simulink model "model"  (R2023a)
settings: Solver=VariableStepAuto  StartTime=0.0  StopTime=0.25  RelTol=1e-3
values from neighbouring files (symbols this model uses):
  Bm = 10^(-5)    (= 1e-05)    [parameter.m]
  g = 9.81    [parameter.m]
  J1 = 1.475*10^(-3)    (= 0.001475)    [parameter.m]
  J2 = 1.155*10^(-4)    (= 0.0001155)    [parameter.m]
  Jm = 3*10^(-5)    (= 3e-05)    [parameter.m]
  Km = 0.0267    [parameter.m]
  L = 5*10^(-3)    (= 0.005)    [parameter.m]
  L1 = 0.05    [parameter.m]
  L2 = 0.08    [parameter.m]
  m1 = 0.7    [parameter.m]
  m2 = 0.25    [parameter.m]
  R = 4    [parameter.m]
settings Model: Creator=USER  LastModifiedBy=USER

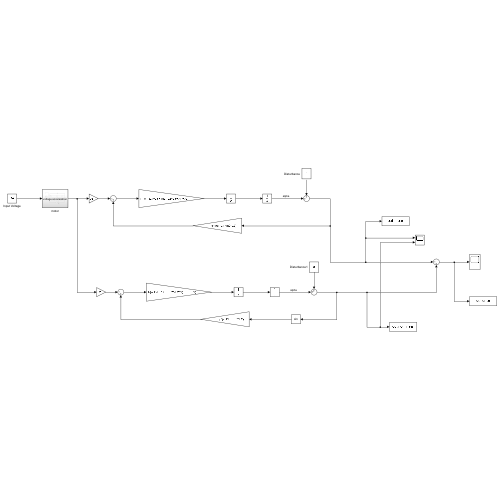
[thumbnail: Simulink's stored preview of the top-level diagram]
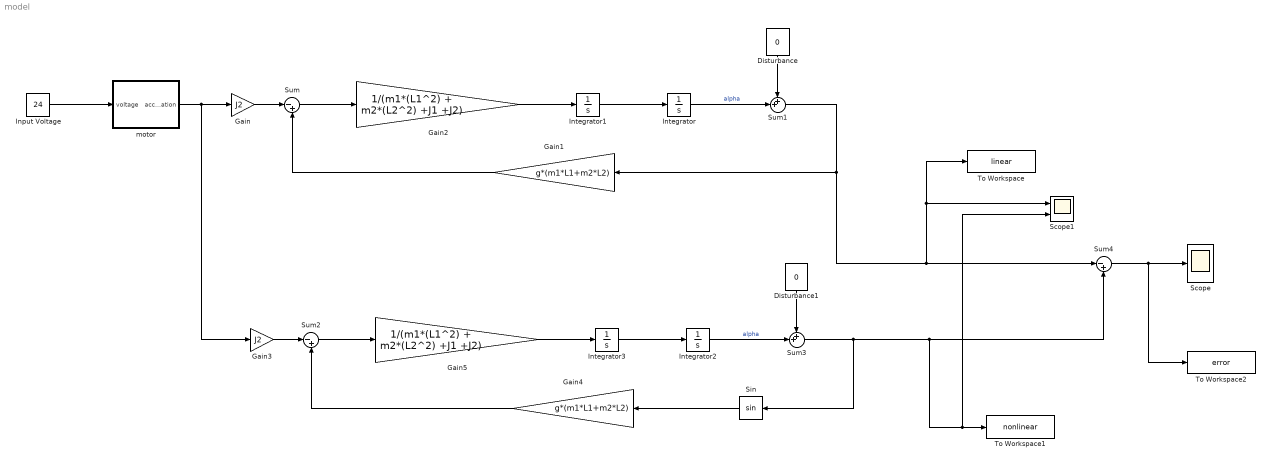
== system model ==
  Disturbance : Constant  Value=0
  Disturbance1 : Constant  Value=0
  Gain : Gain  Gain=J2
  Gain1 : Gain  Gain=g*(m1*L1+m2*L2)
  Gain2 : Gain  Gain=1/(m1*(L1^2) + m2*(L2^2) +J1 +J2)
  Gain3 : Gain  Gain=J2
  Gain4 : Gain  Gain=g*(m1*L1+m2*L2)
  Gain5 : Gain  Gain=1/(m1*(L1^2) + m2*(L2^2) +J1 +J2)
  Input Voltage : Constant  Value=24
  Integrator{,1..3} (4 alike) : Integrator
  Scope : Scope
  Scope1 : Scope  NumInputPorts=2
  Sin : Trigonometry
  Sum : Sum  Inputs=|-+
  Sum1 : Sum  Inputs=++|
  Sum2 : Sum  Inputs=|-+
  Sum3 : Sum  Inputs=++|
  Sum4 : Sum  Inputs=|-+
  To Workspace : ToWorkspace  VariableName=linear  SaveFormat=Timeseries  SampleTime=-1
  To Workspace1 : ToWorkspace  VariableName=nonlinear  SaveFormat=Timeseries  SampleTime=-1
  To Workspace2 : ToWorkspace  VariableName=error  SaveFormat=Timeseries  SampleTime=-1
  motor : Subsystem
  wires:
  Input Voltage/1 -> motor/1(voltage)
  Integrator1/1 -> Integrator/1
  Integrator/1 -> Sum1/2  "alpha"
  motor/1(acceleration) -> Gain3/1, Gain/1
  Gain/1 -> Sum/1
  Gain1/1 -> Sum/2
  Sum/1 -> Gain2/1
  Gain2/1 -> Integrator1/1
  Disturbance/1 -> Sum1/1
  Sum1/1 -> To Workspace/1, Scope1/1, Sum4/1, Gain1/1
  Disturbance1/1 -> Sum3/1
  Gain4/1 -> Sum2/2
  Gain3/1 -> Sum2/1
  Sum2/1 -> Gain5/1
  Gain5/1 -> Integrator3/1
  Integrator3/1 -> Integrator2/1
  Integrator2/1 -> Sum3/2  "alpha"
  Sin/1 -> Gain4/1
  Sum4/1 -> To Workspace2/1, Scope/1
  Sum3/1 -> Scope1/2, To Workspace1/1, Sum4/2, Sin/1

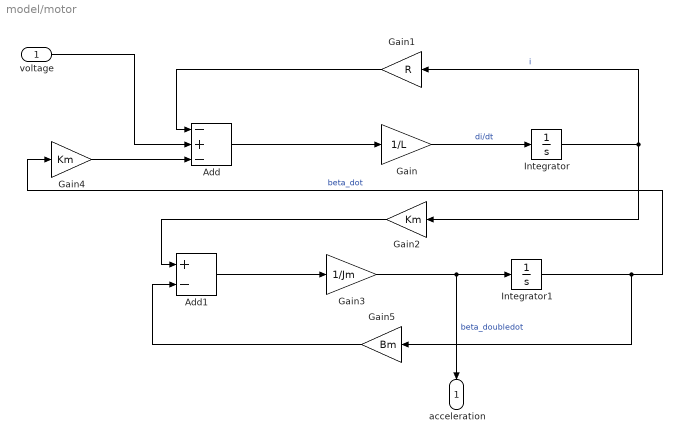
== system model/motor ==
  voltage : Inport
  Add : Sum  Inputs=-+-
  Add1 : Sum  Inputs=+-
  Gain : Gain  Gain=1/L
  Gain1 : Gain  Gain=R
  Gain2 : Gain  Gain=Km
  Gain3 : Gain  Gain=1/Jm
  Gain4 : Gain  Gain=Km
  Gain5 : Gain  Gain=Bm
  Integrator : Integrator
  Integrator1 : Integrator
  acceleration : Outport
  wires:
  Gain/1 -> Integrator/1  "di/dt"
  Integrator1/1 -> Gain5/1, Gain4/1  "beta_dot"
  Gain2/1 -> Add1/1
  Add/1 -> Gain/1
  voltage/1 -> Add/2
  Gain4/1 -> Add/3
  Gain5/1 -> Add1/2
  Integrator/1 -> Gain2/1, Gain1/1  "i"
  Gain1/1 -> Add/1
  Gain3/1 -> acceleration/1, Integrator1/1  "beta_doubledot"
  Add1/1 -> Gain3/1
